simulink model "L6W1_ThreePhaseHBridge"  (R2021a)
settings: Solver=VariableStepAuto  StartTime=0.0  StopTime=0.08  RelTol=1e-3
libraries: spsIGBTDiodeLib x24, spsDCVoltageSourceLib x6, spsTriangleGeneratorLib x6, spsVoltageMeasurementLib x6, spsCurrentMeasurementLib x3, spsSeriesRLCBranchLib x3, spspowerguiLib x1
settings Model: Creator=hp  LastModifiedBy=hp

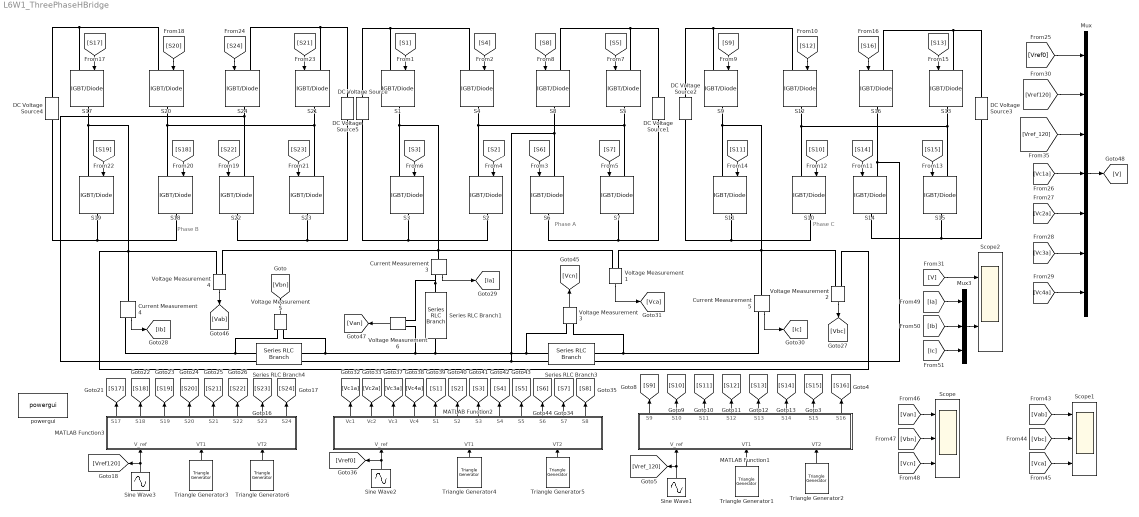
== system L6W1_ThreePhaseHBridge ==
  note: Phase A
  note: Phase B
  note: Phase C
  Current Measurement3 : spsCurrentMeasurementLib/Current Measurement  PhasorSimulation=off  OutputType=Complex  PSBequivalent=0
  Current Measurement4 : spsCurrentMeasurementLib/Current Measurement  PhasorSimulation=off  OutputType=Complex  PSBequivalent=0
  Current Measurement5 : spsCurrentMeasurementLib/Current Measurement  PhasorSimulation=off  OutputType=Complex  PSBequivalent=0
  DC Voltage Source{,1..5} (6 alike) : spsDCVoltageSourceLib/DC Voltage Source  Amplitude=50  Measurements=None
  MATLAB Function1 : MATLAB Function  TreatAsAtomicUnit=on
  MATLAB Function2 : MATLAB Function  TreatAsAtomicUnit=on
  MATLAB Function3 : MATLAB Function  TreatAsAtomicUnit=on
  Mux : Mux  Inputs=7
  Mux3 : Mux  Inputs=3
  S{1..24} (24 alike) : spsIGBTDiodeLib/IGBT//Diode  Ron=1e-3  Rs=1e5  Cs=inf  Measurements=off
  Scope : Scope  NumInputPorts=3
  Scope1 : Scope  NumInputPorts=3
  Scope2 : Scope  NumInputPorts=2
  Series RLC Branch1 : spsSeriesRLCBranchLib/Series RLC Branch  LConnTagsString=__new0  RConnTagsString=__new0  BranchType=RL  Resistance=5  Inductance=100e-3  SetiL0=off  InitialCurrent=0  Capacitance=1e-6  Setx0=off  InitialVoltage=0  Measurements=None
  Series RLC Branch3 : spsSeriesRLCBranchLib/Series RLC Branch  LConnTagsString=__new0  RConnTagsString=__new0  BranchType=RL  Resistance=5  Inductance=100e-3  SetiL0=off  InitialCurrent=0  Capacitance=1e-6  Setx0=off  InitialVoltage=0  Measurements=None
  Series RLC Branch4 : spsSeriesRLCBranchLib/Series RLC Branch  LConnTagsString=__new0  RConnTagsString=__new0  BranchType=RL  Resistance=5  Inductance=100e-3  SetiL0=off  InitialCurrent=0  Capacitance=1e-6  Setx0=off  InitialVoltage=0  Measurements=None
  Sine Wave1 : Sin  Frequency=2*pi*50  Phase=240*(pi/180)  SampleTime=0
  Sine Wave2 : Sin  Frequency=2*pi*50  SampleTime=0
  Sine Wave3 : Sin  Frequency=2*pi*50  Phase=120*(pi/180)  SampleTime=0
  Triangle Generator1 : spsTriangleGeneratorLib/Triangle Generator  Freq=1000  Phase=0  Ts=0
  Triangle Generator2 : spsTriangleGeneratorLib/Triangle Generator  Freq=1000  Phase=180  Ts=0
  Triangle Generator3 : spsTriangleGeneratorLib/Triangle Generator  Freq=1000  Phase=0  Ts=0
  Triangle Generator4 : spsTriangleGeneratorLib/Triangle Generator  Freq=1000  Phase=0  Ts=0
  Triangle Generator5 : spsTriangleGeneratorLib/Triangle Generator  Freq=1000  Phase=180  Ts=0
  Triangle Generator6 : spsTriangleGeneratorLib/Triangle Generator  Freq=1000  Phase=180  Ts=0
  Voltage Measurement{1..6} (6 alike) : spsVoltageMeasurementLib/Voltage Measurement  PhasorSimulation=off  OutputType=Complex  PSBequivalent=0
  powergui : spspowerguiLib/powergui  Priority=1  SimulationMode=Discrete  SampleTime=50e-6  frequency=60  Iterations=50  frequencyindice=0  Pbase=100e6  ErrMax=1e-4  UnitsV=kV  UnitsW=MW  buscounter=0  FunctionMessages=off  echomessages=off  EnableUseOfTLC=off  CurrentSourceSwitches=off  DisableSnubberDevices=off  DisableRonSwitches=off  DisableVfSwitches=off  DisplayEquations=off  AutomaticDiscreteSolvers=off  SolverType=Tustin/Backward Euler (TBE)  Interpol=off  ExternalGateDelay=off  methode=off  Ts=100  x0status=blocks  SPID=on  SwTol=0  HookPort=off  NonlinearTolerance=1e-4  nMaxIteration=100  ContinueOnMaxIteration=off  RestoreLinks=warning  ResistiveCurrentMeasurement=off  Frange=[0:2:500]  Ylog=off  Xlog=on  ShowGrid=off  save=off  variable=ZData  structure=a  ZoomFFT=on  StartTime=0.1  cycles=5  DisplayStyle=1  fundamental=50  FreqAxis=on  MaxFrequency=10000  frequencyindicesteady=1  RmsSteady=1  display=off
  wires:
  [S7] -> S7/1
  [S3] -> S3/1
  [S2] -> S2/1
  [S8] -> S8/1
  [S1] -> S1/1
  [S4] -> S4/1
  [S5] -> S5/1
  [S6] -> S6/1
  Triangle Generator4/1 -> MATLAB Function2/2(VT1)
  MATLAB Function2/2(Vc2) -> [Vc2a]
  Sine Wave2/1 -> MATLAB Function2/1(V_ref), [Vref0]
  MATLAB Function2/1(Vc1) -> [Vc1a]
  MATLAB Function2/7(S3) -> [S3]
  MATLAB Function2/10(S6) -> [S6]
  MATLAB Function2/9(S5) -> [S5]
  MATLAB Function2/5(S1) -> [S1]
  MATLAB Function2/12(S8) -> [S8]
  MATLAB Function2/8(S4) -> [S4]
  MATLAB Function2/11(S7) -> [S7]
  MATLAB Function2/6(S2) -> [S2]
  Triangle Generator5/1 -> MATLAB Function2/3(VT2)
  MATLAB Function2/3(Vc3) -> [Vc3a]
  MATLAB Function2/4(Vc4) -> [Vc4a]
  [S12] -> S12/1
  [S13] -> S13/1
  [S9] -> S9/1
  [S15] -> S15/1
  [S10] -> S10/1
  [S16] -> S16/1
  [S11] -> S11/1
  [S14] -> S14/1
  [S20] -> S20/1
  [S21] -> S21/1
  [S17] -> S17/1
  [S23] -> S23/1
  [S18] -> S18/1
  [S24] -> S24/1
  [S19] -> S19/1
  [S22] -> S22/1
  Triangle Generator2/1 -> MATLAB Function1/3(VT2)
  MATLAB Function1/5(S13) -> [S13]
  MATLAB Function1/8(S16) -> [S16]
  MATLAB Function1/3(S11) -> [S11]
  MATLAB Function1/7(S15) -> [S15]
  MATLAB Function1/4(S12) -> [S12]
  MATLAB Function1/1(S9) -> [S9]
  MATLAB Function1/2(S10) -> [S10]
  Triangle Generator1/1 -> MATLAB Function1/2(VT1)
  MATLAB Function1/6(S14) -> [S14]
  Sine Wave1/1 -> MATLAB Function1/1(V_ref), [Vref_120]
  Triangle Generator6/1 -> MATLAB Function3/3(VT2)
  MATLAB Function3/5(S21) -> [S21]
  MATLAB Function3/8(S24) -> [S24]
  MATLAB Function3/3(S19) -> [S19]
  MATLAB Function3/7(S23) -> [S23]
  MATLAB Function3/4(S20) -> [S20]
  MATLAB Function3/1(S17) -> [S17]
  MATLAB Function3/2(S18) -> [S18]
  Triangle Generator3/1 -> MATLAB Function3/2(VT1)
  MATLAB Function3/6(S22) -> [S22]
  Sine Wave3/1 -> MATLAB Function3/1(V_ref), [Vref120]
  Voltage Measurement2/1 -> [Vbc]
  Current Measurement5/1 -> [Ic]
  Voltage Measurement1/1 -> [Vca]
  Voltage Measurement3/1 -> [Vcn]
  Current Measurement3/1 -> [Ia]
  Voltage Measurement5/1 -> [Vbn]
  Current Measurement4/1 -> [Ib]
  Voltage Measurement4/1 -> [Vab]
  Voltage Measurement6/1 -> [Van]
  [Vref0] -> Mux/1
  Mux/1 -> [V]
  [Ia] -> Mux3/1
  [Ib] -> Mux3/2
  [Ic] -> Mux3/3
  [Van] -> Scope/1
  [Vbn] -> Scope/2
  [Vcn] -> Scope/3
  [Vab] -> Scope1/1
  [Vbc] -> Scope1/2
  [Vca] -> Scope1/3
  [Vc4a] -> Mux/7
  [Vc3a] -> Mux/6
  [Vc2a] -> Mux/5
  [Vc1a] -> Mux/4
  [Vref_120] -> Mux/3
  [Vref120] -> Mux/2
  Mux3/1 -> Scope2/2
  [V] -> Scope2/1
  connections:
  S7/RConn1 -- DC Voltage Source1/LConn1 -- S6/RConn1
  S8/LConn1 -- DC Voltage Source1/RConn1 -- S5/LConn1
  S7/LConn1 -- S4/RConn1 -- S2/LConn1 -- S5/RConn1
  S3/LConn1 -- Voltage Measurement4/LConn1 -- Voltage Measurement1/LConn2 -- Current Measurement3/LConn1 -- S1/RConn1
  DC Voltage Source/LConn1 -- S2/RConn1 -- S3/RConn1
  DC Voltage Source/RConn1 -- S4/LConn1 -- S1/LConn1
  Series RLC Branch3/RConn1 -- S14/LConn1 -- S16/RConn1 -- S22/LConn1 -- S24/RConn1 -- S8/RConn1 -- S6/LConn1 -- Series RLC Branch1/RConn1 -- Voltage Measurement6/LConn2 -- Series RLC Branch4/RConn1 -- Voltage Measurement5/LConn2 -- Voltage Measurement3/LConn2
  Current Measurement3/RConn1 -- Voltage Measurement6/LConn1 -- Series RLC Branch1/LConn1
  S9/LConn1 -- S12/LConn1 -- DC Voltage Source2/RConn1
  S11/RConn1 -- DC Voltage Source2/LConn1 -- S10/RConn1
  DC Voltage Source3/LConn1 -- S15/RConn1 -- S14/RConn1
  S9/RConn1 -- Voltage Measurement1/LConn1 -- Voltage Measurement2/LConn2 -- Current Measurement5/LConn1 -- S11/LConn1
  S13/LConn1 -- DC Voltage Source3/RConn1 -- S16/LConn1
  S15/LConn1 -- S13/RConn1 -- S12/RConn1 -- S10/LConn1
  S17/LConn1 -- DC Voltage Source4/RConn1 -- S20/LConn1
  S19/RConn1 -- DC Voltage Source4/LConn1 -- S18/RConn1
  S23/RConn1 -- DC Voltage Source5/LConn1 -- S22/RConn1
  S17/RConn1 -- Voltage Measurement2/LConn1 -- Voltage Measurement4/LConn2 -- Current Measurement4/LConn1 -- S19/LConn1
  DC Voltage Source5/RConn1 -- S21/LConn1 -- S24/LConn1
  S23/LConn1 -- S20/RConn1 -- S18/LConn1 -- S21/RConn1
  Current Measurement4/RConn1 -- Voltage Measurement5/LConn1 -- Series RLC Branch4/LConn1
  Current Measurement5/RConn1 -- Voltage Measurement3/LConn1 -- Series RLC Branch3/LConn1

== matlab function L6W1_ThreePhaseHBridge/MATLAB Function1 ==
  data: V_ref input; VT1 input; VT2 input; S9 output; S10 output; S11 output; S12 output; S13 output; S14 output; S15 output; S16 output
function [S9,S10,S11,S12,S13,S14,S15,S16]= fcn(V_ref,VT1,VT2)
Vc2 = (VT1+1)*.25
Vc1 = ((VT1+3)*.25)
Vc3 = (VT2-1)*.25
Vc4 = ((VT2-3)*.25)
if V_ref>0
    if V_ref>=0 && V_ref<0.5 
        if V_ref>=Vc2
            S9=1;    S10=1;    S11=0;    S12=0;
            S13=0;    S14=1;    S15=1;    S16=0;
        else
            S9=1;    S10=0;    S11=0;    S12=1;
            S13=1;    S14=0;    S15=0;    S16=1;
        end
    else V_ref>=0.5
        if V_ref>=Vc1
            S9=1;    S10=1;    S11=0;    S12=0;
            S13=1;    S14=1;    S15=0;    S16=0;
        else   
            S9=1;    S10=1;    S11=0;    S12=0;
            S13=1;    S14=0;    S15=0;    S16=1;
       end
    end
else
    if V_ref<0 && V_ref>=-0.5
        if V_ref<Vc3      
            S9=1;    S10=0;    S11=0;    S12=1;
            S13=0;    S14=0;    S15=1;    S16=1;
        else
            S9=1;    S10=0;    S11=0;    S12=1;
            S13=1;    S14=0;    S15=0;    S16=1;
        end
    else V_ref<=-0.5
        if V_ref<Vc4       
            S9=0;    S10=0;    S11=1;    S12=1;
            S13=0;    S14=0;    S15=1;    S16=1;
        else         
            S9=0;    S10=0;    S11=1;    S12=1;
            S13=1;    S14=0;    S15=0;    S16=1;
        end        
    end    
end
end

== matlab function L6W1_ThreePhaseHBridge/MATLAB Function3 ==
  data: V_ref input; VT1 input; VT2 input; S17 output; S18 output; S19 output; S20 output; S21 output; S22 output; S23 output; S24 output
function [S17,S18,S19,S20,S21,S22,S23,S24]= fcn(V_ref,VT1,VT2)
Vc2 = (VT1+1)*.25
Vc1 = ((VT1+3)*.25)
Vc3 = (VT2-1)*.25
Vc4 = ((VT2-3)*.25)
if V_ref>0
    if V_ref>=0 && V_ref<0.5 
        if V_ref>=Vc2
            S17=1;    S18=1;    S19=0;    S20=0;
            S21=0;    S22=1;    S23=1;    S24=0;
        else
            S17=1;    S18=0;    S19=0;    S20=1;
            S21=1;    S22=0;    S23=0;    S24=1;
        end
    else V_ref>=0.5
        if V_ref>=Vc1
            S17=1;    S18=1;    S19=0;    S20=0;
            S21=1;    S22=1;    S23=0;    S24=0;
        else   
            S17=1;    S18=1;    S19=0;    S20=0;
            S21=1;    S22=0;    S23=0;    S24=1;
       end
    end
else
    if V_ref<0 && V_ref>=-0.5
        if V_ref<Vc3      
            S17=1;    S18=0;    S19=0;    S20=1;
            S21=0;    S22=0;    S23=1;    S24=1;
        else
            S17=1;    S18=0;    S19=0;    S20=1;
            S21=1;    S22=0;    S23=0;    S24=1;
        end
    else V_ref<=-0.5
        if V_ref<Vc4       
            S17=0;    S18=0;    S19=1;    S20=1;
            S21=0;    S22=0;    S23=1;    S24=1;
        else         
            S17=0;    S18=0;    S19=1;    S20=1;
            S21=1;    S22=0;    S23=0;    S24=1;
        end        
    end    
end
end

== matlab function L6W1_ThreePhaseHBridge/MATLAB Function2 ==
  data: V_ref input; Vc1 output; VT1 input; VT2 input; Vc2 output; Vc3 output; Vc4 output; S1 output; S2 output; S3 output; S4 output; S5 output; S6 output; S7 output; S8 output
function [Vc1,Vc2,Vc3,Vc4,S1,S2,S3,S4,S5,S6,S7,S8]= fcn(V_ref,VT1,VT2)
Vc2 = (VT1+1)*.25
Vc1 = ((VT1+3)*.25)
Vc3 = (VT2-1)*.25
Vc4 = ((VT2-3)*.25)
if V_ref>0
    if V_ref>=0 && V_ref<0.5 
        if V_ref>=Vc2
            S1=1;    S2=1;    S3=0;    S4=0;
            S5=0;    S6=1;    S7=1;    S8=0;
        else
            S1=1;    S2=0;    S3=0;    S4=1;
            S5=1;    S6=0;    S7=0;    S8=1;
        end
    else V_ref>=0.5
        if V_ref>=Vc1
            S1=1;    S2=1;    S3=0;    S4=0;
            S5=1;    S6=1;    S7=0;    S8=0;
        else   
            S1=1;    S2=1;    S3=0;    S4=0;
            S5=1;    S6=0;    S7=0;    S8=1;
       end
    end
else
    if V_ref<0 && V_ref>=-0.5
        if V_ref<Vc3      
            S1=1;    S2=0;    S3=0;    S4=1;
            S5=0;    S6=0;    S7=1;    S8=1;
        else
            S1=1;    S2=0;    S3=0;    S4=1;
            S5=1;    S6=0;    S7=0;    S8=1;
        end
    else V_ref<=-0.5
        if V_ref<Vc4       
            S1=0;    S2=0;    S3=1;    S4=1;
            S5=0;    S6=0;    S7=1;    S8=1;
        else         
            S1=0;    S2=0;    S3=1;    S4=1;
            S5=1;    S6=0;    S7=0;    S8=1;
        end        
    end    
end
end
